simulink model "rotor_control_MOPPC"  (R2016a)
settings: Solver=VariableStepAuto  StartTime=0.0  StopTime=30  RelTol=1e-3
undefined symbols (not defined in the file or in its folder): load_amp, load_finish, load_start, measurement_variance, pulse_period, ref_amp, ref_mean, rotor_h, sinusoid_frequency
settings Model: Creator=Daniel  LastModifiedBy=mgreiff
settings DataIOCC: LimitDataPoints=on
settings DebuggingCC: AllowSymbolicDim=off
settings ModelReferenceCC: PropagateSignalLabelsOutOfModel=off
settings GRTTargetCC: GeneratePreprocessorConditionals=Use local settings

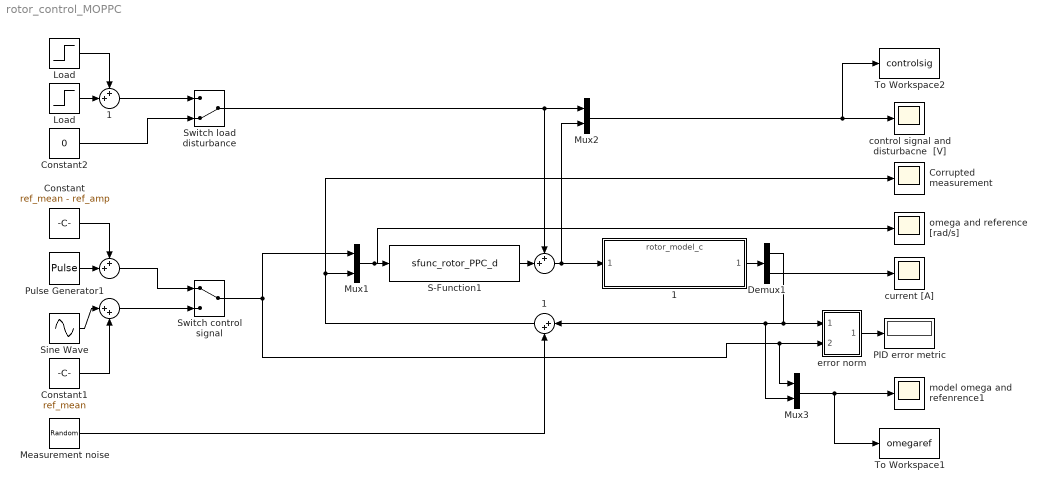
== system rotor_control_MOPPC ==
  " " : Sum  Inputs=++|
  "      " : Sum  Inputs=++|
  "       " : Sum  Inputs=|++
  "       1" : Sum  Inputs=|++
  "      1" : Sum  Inputs=++|
  "   1" : ModelReference  ModelNameDialog=rotor_model_c.slx  SimulationMode=Normal  ModelReferenceVersion=1.30
  " omega and reference [rad/s]" : Scope
  Constant : Constant  Value=ref_mean - ref_amp
  Constant1 : Constant  Value=ref_mean
  Constant2 : Constant  Value=0
  Corrupted measurement : Scope
  Demux1 : Demux  Outputs=2
  Load : Step  Time=load_finish  After=-load_amp  SampleTime=0
  "Load " : Step  Time=load_start  After=load_amp  SampleTime=0
  Measurement noise : RandomNumber  Variance=measurement_variance  SampleTime=rotor_h
  Mux1 : Mux  Inputs=2
  Mux2 : Mux  Inputs=2
  Mux3 : Mux  Inputs=2
  PID error metric : Display
  Pulse Generator1 : DiscretePulseGenerator  PulseType=Time based  Amplitude=ref_amp*2  Period=pulse_period  PulseWidth=50
  S-Function1 : S-Function  FunctionName=sfunc_rotor_PPC_d  Parameters=MOPPCparam  SFunctionDeploymentMode=off  EnableBusSupport=off
  Sine Wave : Sin  Amplitude=200  Frequency=sinusoid_frequency  SampleTime=0
  Switch control signal : ManualSwitch
  Switch load disturbance : ManualSwitch  CurrentSetting=0
  To Workspace1 : ToWorkspace  VariableName=omegaref  SaveFormat=Timeseries  SampleTime=-1
  To Workspace2 : ToWorkspace  VariableName=controlsig  SaveFormat=Timeseries  SampleTime=-1
  control signal and disturbacne  [V] : Scope
  "current [A]   " : Scope
  error norm : Subsystem
  model omega and refenrence1 : Scope
  wires:
  "   1"/1 -> Demux1/1
  Constant/1 -> "      "/1
  Demux1/2 -> "current [A]   "/1
  "      "/1 -> Switch control signal/1
  Pulse Generator1/1 -> "      "/2
  Sine Wave/1 -> "       "/1
  "       "/1 -> Switch control signal/2
  Constant1/1 -> "       "/2
  " "/1 -> "   1"/1, Mux2/2
  Mux1/1 -> " omega and reference [rad/s]"/1, S-Function1/1
  Switch load disturbance/1 -> " "/1, Mux2/1
  Mux2/1 -> To Workspace2/1, control signal and disturbacne  [V]/1
  Switch control signal/1 -> error norm/2(In2), Mux3/1, Mux1/1
  Mux3/1 -> model omega and refenrence1/1, To Workspace1/1
  "Load "/1 -> "      1"/1
  Load/1 -> "      1"/2
  error norm/1(Out1) -> PID error metric/1
  "      1"/1 -> Switch load disturbance/1
  Constant2/1 -> Switch load disturbance/2
  Demux1/1 -> "       1"/1, Mux3/2, error norm/1(In1)
  "       1"/1 -> Mux1/2, Corrupted measurement/1
  Measurement noise/1 -> "       1"/2
  S-Function1/1 -> " "/2

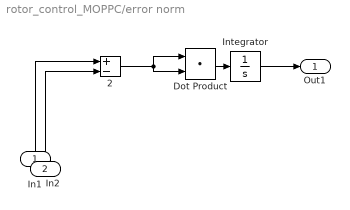
== system rotor_control_MOPPC/error norm ==
  In1 : Inport
  In2 : Inport  Port=2
  "      2" : Sum  Inputs=+-
  Dot Product : DotProduct  InputSameDT=on  OutDataTypeStr=Inherit: Inherit via internal rule
  Integrator : Integrator
  Out1 : Outport
  wires:
  "      2"/1 -> Dot Product/1, Dot Product/2
  Dot Product/1 -> Integrator/1
  In1/1 -> "      2"/1
  In2/1 -> "      2"/2
  Integrator/1 -> Out1/1
